simulink model "Sec3_Step_1_FORC_Experiment"  (R2020a)
settings: Solver=ode4  StartTime=0.0  StopTime=20.0  FixedStep=.0001  MaxStep=1e-4  RelTol=1e-3
settings Model: Creator=nnnmmm  LastModifiedBy=nnnmmm
settings DataIOCC: ExternalInput=sim_input_T

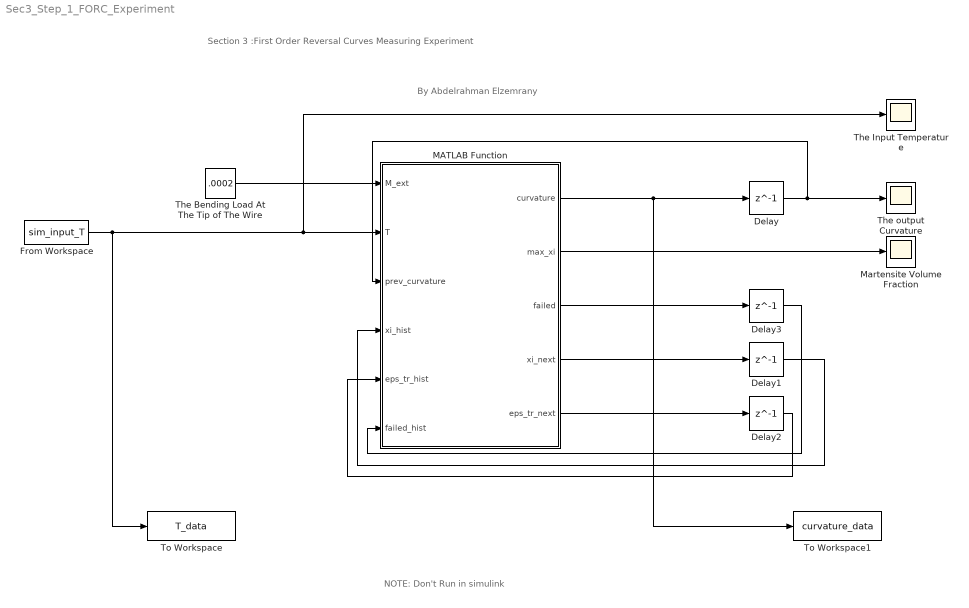
== system Sec3_Step_1_FORC_Experiment ==
  note: NOTE: Don't Run in simulink
  note: By Abdelrahman Elzemrany
  note: Section 3 :First Order Reversal Curves Measuring Experiment
  Delay : Delay  DelayLength=1
  Delay1 : Delay  DelayLength=1  InitialCondition=ones(1,11)
  Delay2 : Delay  DelayLength=1  InitialCondition=zeros(1,11)
  Delay3 : Delay  DelayLength=1
  From Workspace : FromWorkspace  VariableName=sim_input_T
  MATLAB Function : MATLAB Function  TreatAsAtomicUnit=on
  Martensite Volume Fraction : Scope
  The Bending Load At The Tip of The Wire : Constant  Value=.0002
  The Input Temperature : Scope
  The output Curvature : Scope
  To Workspace : ToWorkspace  VariableName=T_data  SaveFormat=Timeseries  SampleTime=-1
  To Workspace1 : ToWorkspace  VariableName=curvature_data  SaveFormat=Timeseries  SampleTime=-1
  wires:
  Delay2/1 -> MATLAB Function/5(eps_tr_hist)
  MATLAB Function/5(eps_tr_next) -> Delay2/1
  MATLAB Function/1(curvature) -> Delay/1, To Workspace1/1
  MATLAB Function/3(failed) -> Delay3/1
  MATLAB Function/4(xi_next) -> Delay1/1
  Delay/1 -> MATLAB Function/3(prev_curvature), The output Curvature/1
  Delay3/1 -> MATLAB Function/6(failed_hist)
  Delay1/1 -> MATLAB Function/4(xi_hist)
  The Bending Load At The Tip of The Wire/1 -> MATLAB Function/1(M_ext)
  MATLAB Function/2(max_xi) -> Martensite Volume Fraction/1
  From Workspace/1 -> To Workspace/1, The Input Temperature/1, MATLAB Function/2(T)

== matlab function Sec3_Step_1_FORC_Experiment/MATLAB Function ==
  data: M_ext input; T input; prev_curvature input; xi_hist input; eps_tr_hist input; curvature output; max_xi output; failed_hist input; failed output; xi_next output; eps_tr_next output
function [curvature, max_xi,  failed, xi_next, eps_tr_next] = lagoudas_wire_pure_bending(M_ext , T, prev_curvature, xi_hist, eps_tr_hist, failed_hist)
%#codegen

% =========================================================================
% ─── SIMULINK CODER INCLUSIONS: IMMEDIATE VARIABLE INITIALIZATION ───
% =========================================================================
failed = failed_hist; % FIX: Inherit historical failure state immediately
curvature = prev_curvature;
max_xi = 0.0;


% Strict [11 x 1] column vector properties for code generation alignment
xi_next = zeros(11, 1);
eps_tr_next = zeros(11, 1);

% Early exit if the wire has already failed historically
if failed_hist > 0.5
    failed = 1.0;
    return;
end

% =========================================================================
% 1. WIRE CROSS-SECTIONAL SLICE DISCRETIZATION (11 Symmetrical Layers)
% =========================================================================
R_wire = 0.25e-3;   
N_layers = 11;      
y_coords = linspace(-R_wire, R_wire, N_layers); 
y_coords = y_coords(:); 
dy = y_coords(2) - y_coords(1);
dt = 0.0001;        

xi_current = xi_hist(:);
eps_tr_current = eps_tr_hist(:);

% =========================================================================
% 2. EXPLICIT MATERIAL LITERAL CONSTANTS
% =========================================================================
E_A = 70e9;             
E_M = 30e9;             
H_max = 0.045;          
sigma_failure = 1000e6; 

Ms = 275; Mf = 256; As = 280; Af = 300; % Ms updated to 280 K
C_A = 8e6; C_M = 8e6;   
n1 = 2.0; n2 = 2.0; n3 = 2.0; n4 = 2.0; 

S_A = 1 / E_A; S_M = 1 / E_M; Delta_S = S_M - S_A; 

w_layer = 2 * sqrt(max(0, R_wire^2 - y_coords.^2));
dA = w_layer * dy;
S_curr_static = S_A + xi_current * Delta_S;

% =========================================================================
% 3. VECTORIZED EXPLICIT STATIC SOLVER LOOP FOR MECHANICAL EQUILIBRIUM
% =========================================================================
low_k = -150.0; 
high_k = 150.0; 
tol = 1e-6;
curvature = prev_curvature;
residual_mid = 0.0;

for iter = 1:60
    mid_k = (low_k + high_k) / 2;
    
    % Evaluate midpoint state residual
    eps_mid = -y_coords * mid_k;
    sigma_mid = (eps_mid - eps_tr_current) ./ S_curr_static;
    M_calc_mid = sum(-sigma_mid .* y_coords .* dA);
    residual_mid = M_calc_mid - M_ext;
    
    % Evaluate low-point state residual dynamically inside the loop
    % FIX: This forces the boundary checks to update with each step
    eps_low = -y_coords * low_k;
    sigma_low = (eps_low - eps_tr_current) ./ S_curr_static;
    M_calc_low = sum(-sigma_low .* y_coords .* dA);
    residual_low = M_calc_low - M_ext;
    
    if abs(residual_mid) < tol
        curvature = mid_k;
        break;
    end
    
    if (residual_low * residual_mid) < 0
        high_k = mid_k;
    else
        low_k = mid_k;
    end
end

if abs(residual_mid) >= tol
    curvature = (low_k + high_k) / 2;
end

% =========================================================================
% 4. LAYER PROGRESSION UPDATE WITH EXPLICIT RELAXATION FILTERING
% =========================================================================
sigma_max_track = 0.0;
xi_unfiltered = zeros(N_layers, 1);

for j = 1:N_layers
    epsilon = -y_coords(j) * curvature;
    S_curr = S_A + xi_current(j) * Delta_S;
    sigma_layer = (epsilon - eps_tr_current(j)) / S_curr;
    
    if abs(sigma_layer) > sigma_max_track
        sigma_max_track = abs(sigma_layer);
    end
    
    sgn_sig = sign(sigma_layer);
    if sgn_sig == 0; sgn_sig = 1; end
    
    Ms_s = Ms + abs(sigma_layer) / C_M;
    Mf_s = Mf + abs(sigma_layer) / C_M;
    As_s = As + abs(sigma_layer) / C_A;
    Af_s = Af + abs(sigma_layer) / C_A;
    
    xi_target = xi_current(j); 
    
    if abs(curvature) > 0.005
        if (T < Ms_s) && (T > Mf_s)
            linear_ratio = (T - Mf_s) / (Ms_s - Mf_s);
            trial_target = 1.0 - (linear_ratio^n1 / (linear_ratio^n1 + (1.0 - linear_ratio)^n2));
            if trial_target > xi_current(j); xi_target = trial_target; end
        elseif T <= Mf_s
            xi_target = 1.0;
        end
        
        if (T > As_s) && (T < Af_s)
            linear_ratio = (T - As_s) / (Af_s - As_s);
            trial_target = 1.0 - (linear_ratio^n3 / (linear_ratio^n3 + (1.0 - linear_ratio)^n4));
            if trial_target < xi_current(j); xi_target = trial_target; end
        elseif T >= Af_s
            xi_target = 0.0;
        end
    else
        if T > Af; xi_target = 0.0; elseif T < Mf; xi_target = 1.0; end
    end
    
    xi_unfiltered(j) = xi_target;
    
    % Balanced 5% relaxation factor
    xi_current(j) = xi_hist(j) + 0.05 * (xi_target - xi_hist(j));
    
    sigma_detwin = 70e6;
    if abs(sigma_layer) > 1e-3
        detwin_factor = min(1.0, abs(sigma_layer) / sigma_detwin);
        eps_tr_target = sgn_sig * H_max * xi_current(j) * detwin_factor;
    else
        eps_tr_target = 0.0;
    end
    
    eps_tr_current(j) = eps_tr_hist(j) + 0.05 * (eps_tr_target - eps_tr_hist(j));
end

if sigma_max_track > sigma_failure
    failed = 1.0;
end

% =========================================================================
% 5. ASSIGN FINAL OUTPUT PARAMETERS
% =========================================================================
max_xi = max(xi_current);
surface_sigma = sigma_max_track;

mean_xi_target = mean(xi_unfiltered);
mean_xi_hist = mean(xi_hist);
dxi_dt = (mean_xi_target - mean_xi_hist) / dt;

xi_next = xi_current(:);
eps_tr_next = eps_tr_current(:);

end
